simulink subsystem "BatteryHV_Inputs_Charge_refsub"  (R2025a)
settings: Solver=VariableStepAuto  StartTime=0.0  StopTime=10.0  RelTol=1e-3
undefined symbols (not defined in the file or in its folder): batteryHV, testParam
settings Model: Creator=isaacito  LastModifiedBy=isaacito
settings OptimizationCC: ReuseModelBlockBuffer=off
settings RTWCC: GPUComputeCapability=3.5

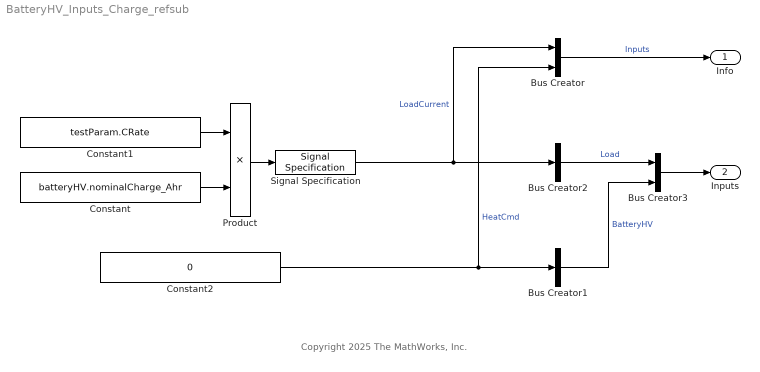
== system BatteryHV_Inputs_Charge_refsub ==
  note: Copyright 2025 The MathWorks, Inc.
  Bus Creator : BusCreator  Inputs=2
  Bus Creator1 : BusCreator  Inputs=1
  Bus Creator2 : BusCreator  Inputs=1
  Bus Creator3 : BusCreator  Inputs=2
  Constant : Constant  Value=batteryHV.nominalCharge_Ahr
  Constant1 : Constant  Value=testParam.CRate
  Constant2 : Constant  Value=0
  Product : Product
  Signal Specification : SignalSpecification  Unit=A
  Info : Outport
  Inputs : Outport  Port=2
  wires:
  Bus Creator/1 -> Info/1  "Inputs"
  Product/1 -> Signal Specification/1
  Bus Creator1/1 -> Bus Creator3/2  "BatteryHV"
  Bus Creator2/1 -> Bus Creator3/1  "Load"
  Bus Creator3/1 -> Inputs/1
  Constant2/1 -> Bus Creator1/1, Bus Creator/2  "HeatCmd"
  Constant1/1 -> Product/1
  Constant/1 -> Product/2
  Signal Specification/1 -> Bus Creator2/1, Bus Creator/1  "LoadCurrent"
